simulink model "simulink_ros"  (R2022b)
settings: Solver=FixedStepAuto  StartTime=0.0  StopTime=setup.stop_time  FixedStep=setup.sim_ts  RelTol=1e-3
InitFcn:
  | %INIT_COSIM
StartFcn:
  | unix('source /home/pico/Documents/GitHub/bfmc/Simulator/devel/setup.bash; rosservice call /gazebo/reset_simulation');
undefined symbols (not defined in the file): nmpc_controller, setup
libraries: robotlib x5, simulink x2
settings Model: Creator=pico  LastModifiedBy=pico

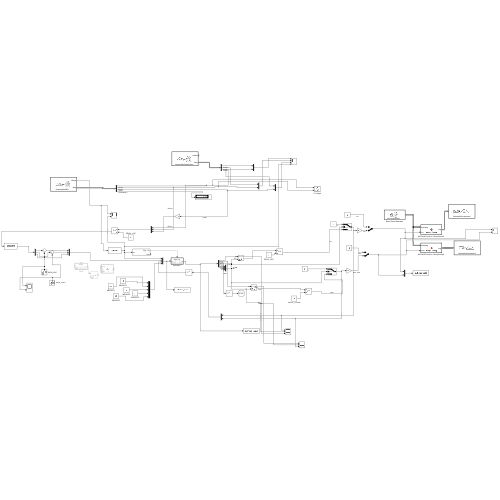
[thumbnail: Simulink's stored preview of the top-level diagram]
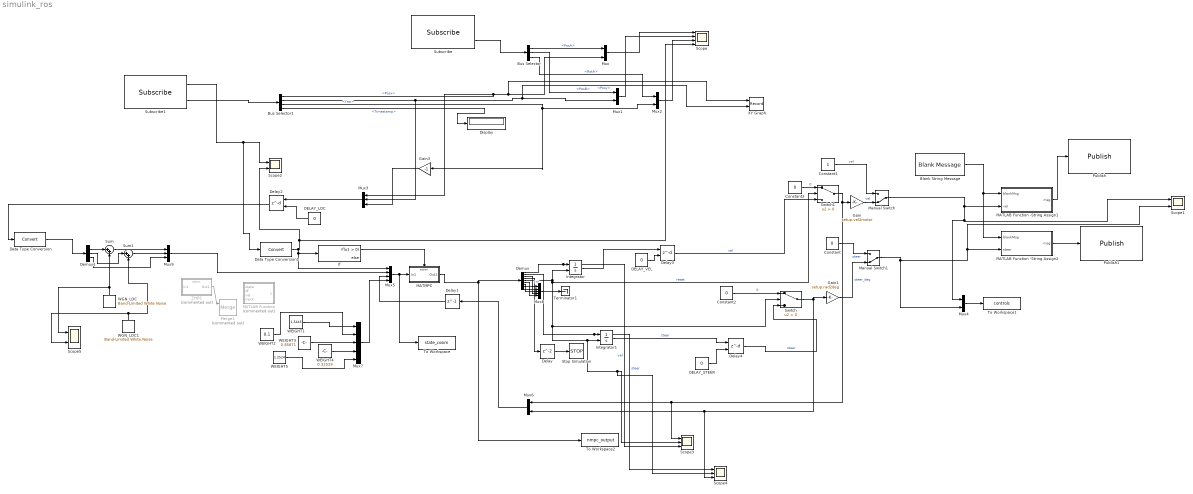
== system simulink_ros ==
  Blank String Message : robotlib/Blank Message  messageClass=Message  entityType=std_msgs/String  messageType=std_msgs/String  SampleTime=inf  legacyBusStruct=off
  Bus Selector : BusSelector  OutputSignals=PosA,PosB,RotA
  Bus Selector1 : BusSelector  OutputSignals=Posx,Posy,Yaw,Timestamp
  Constant : Constant  Value=0
  Constant1 : Constant
  Constant2 : Constant  Value=0
  Constant3 : Constant  Value=0
  DELAY_LOC : Constant  Value=0
  DELAY_STEER : Constant  Value=0
  DELAY_VEL : Constant  Value=0
  Data Type Conversion : DataTypeConversion  SaturateOnIntegerOverflow=off  RndMeth=Floor
  Data Type Conversion1 : DataTypeConversion  SaturateOnIntegerOverflow=off  RndMeth=Floor
  Delay : Delay
  Delay1 : Delay  DelayLength=1
  Delay2 : Delay  DelayLengthSource=Input port  DelayLength=0
      settings: InputPortMap=u0,p1
  Delay3 : Delay  DelayLengthSource=Input port  DelayLength=0
      settings: InputPortMap=u0,p1
  Delay4 : Delay  DelayLengthSource=Input port  DelayLength=0
      settings: InputPortMap=u0,p1
  Demux : Demux  Outputs=9
  Demux1 : Demux  Outputs=3
  Display : Display
  Gain : Gain  Gain=setup.vel2motor
  Gain1 : Gain  Gain=setup.rad2deg
  Gain3 : Gain  Gain=-1
  If : If
  Integrator : Integrator  ExternalReset=level  LimitOutput=on  UpperSaturationLimit=2  LowerSaturationLimit=0
  Integrator1 : Integrator  ExternalReset=level  LimitOutput=on  UpperSaturationLimit=pi/3  LowerSaturationLimit=-pi/3
  MATLAB Function : MATLAB Function  Commented=on  TreatAsAtomicUnit=on
  MATLAB Function -String Assign1 : MATLAB Function  TreatAsAtomicUnit=on
  MATLAB Function -String Assign2 : MATLAB Function  TreatAsAtomicUnit=on
  MATMPC : Subsystem  TreatAsAtomicUnit=on
  Manual Switch : ManualSwitch  CurrentSetting=0
  Manual Switch1 : ManualSwitch  CurrentSetting=0
  Merge1 : Merge  Commented=on
  Mux{,1..2,4,6} (5 alike) : Mux  Inputs=2
  Mux3 : Mux  Inputs=3
  Mux5 : Mux
  Mux7 : Mux  Inputs=5
  Mux8 : Mux  Inputs=5
  Mux9 : Mux  Inputs=3
  Publish : robotlib/Publish  topicSource=Select from ROS network  topic=/automobile/command  messageType=std_msgs/String  legacyBusStruct=off  messageQueueLength=1
      settings: LibrarySourceBlock=roslib/ROS/Publish
  Publish1 : robotlib/Publish  topicSource=Select from ROS network  topic=/automobile/command  messageType=std_msgs/String  legacyBusStruct=off  messageQueueLength=1
      settings: LibrarySourceBlock=roslib/ROS/Publish
  Scope : Scope  NumInputPorts=4
  Scope1 : Scope  NumInputPorts=2
  Scope2 : Scope  NumInputPorts=2
  Scope3 : Scope  NumInputPorts=3
  Scope4 : Scope  NumInputPorts=3
  Scope5 : Scope  NumInputPorts=2
  Stop Simulation : Stop
  Subscribe : robotlib/Subscribe  topicSource=Select from ROS network  topic=/automobile/localisation  messageType=utils/localisation  SampleTime=-1  legacyBusStruct=off  messageQueueLength=1
      settings: LibrarySourceBlock=roslib/ROS/Subscribe
  Subscribe1 : robotlib/Subscribe  topicSource=Select from ROS network  topic=/automobile/IMU  messageType=utils/IMU  SampleTime=-1  legacyBusStruct=off  messageQueueLength=1
      settings: LibrarySourceBlock=roslib/ROS/Subscribe
  Sum : Sum  Inputs=|++
  Sum1 : Sum  Inputs=|++
  Switch : Switch  Criteria=u2 > Threshold  SaturateOnIntegerOverflow=off  InputSameDT=off
  Switch1 : Switch  Criteria=u2 > Threshold  SaturateOnIntegerOverflow=off  InputSameDT=off
  Terminator1 : Terminator
  To Workspace : ToWorkspace  VariableName=state_cosim  SaveFormat=Structure With Time  SampleTime=-1
  To Workspace1 : ToWorkspace  VariableName=controls  SaveFormat=Structure With Time  SampleTime=-1
  To Workspace2 : ToWorkspace  VariableName=nmpc_output  SaveFormat=Structure With Time  SampleTime=-1
  WEIGHT1 : Constant  Value=1.5445
  WEIGHT2 : Constant  Value=0.1
  WEIGHT3 : Constant  Value=0.85671
  WEIGHT4 : Constant  Value=0.32529
  WEIGHT5 : Constant  Value=1.2524
  WGN_LOC : simulink/Sources/Band-Limited White Noise  Cov=WGN_LOC_PWR  Ts=setup.sim_ts  seed=[23341]
  WGN_LOC1 : simulink/Sources/Band-Limited White Noise  Cov=WGN_LOC_PWR  Ts=setup.sim_ts  seed=[23345]
  XY Graph : Record  FileSettingsInternal="{\"entries\":[{\"content\":{\"excelSettings\":{\"content\":{},\"type\":\"Streamout.ExcelSettings\"}},\"type\":\"Streamout.FileSettingStorage\",\"uuid\":\"7e36053c-6d87-4ba8-b961-ab87f153ee78\"}],\"packageUris\":[\"http://schema.mathworks.com/mf0/streamout_blocks/R2020a\"],\"version\":\"1.0\"}"  Layout=[1 1]  SignalsInternal="{\"entries\":[{\"content\":{\"signals\":[{\"content\":{\"blockPath\":[\"simulink_ros/XY Graph\"],\"channel\":[],\"dimensions\":[1],\"domain\":\"simulink_ros/XY Graph\",\"lineColor\":\"#a2142f\",\"plots\":[1],\"port\":1,\"sid\":[\"\"],\"signalID\":1424408,\"signalName\":\"<Posx>\"},\"type\":\"RecordBlkView.Signal\",\"uuid\":\"8700aef8-5ad9-478a-92a4-92141e58aa95\"},{\"content\":{\"blockPath\":[\"simulink_ros/XY Graph\"],\"channel\":[],\"dimensions\":[1],\"domain\":\"simulink_ros/XY Graph\",\"lineColor\":\"#139fff\",\"plots\":[1],\"port\":2,\"sid\":[\"\"],\"signalID\":1424412,\"signalName\":\"<Posy>\"},\"type\":\"RecordBlkView.Signal\",\"uuid\":\"c04be6e4-d870-4e8a-b9da-b27d68976f23\"}]},\"type\":\"RecordBlkView.InputSignals\",\"uuid\":\"eb864215-60c0-44ea-aa5a-99772fb5c421\"}],\"packageUris\":[\"http://schema.mathworks.com/mf0/streamout_blocks/R2020a\"],\"version\":\"1.0\"}"  VisualizationBindings="{\"xyplotplugin\":{\"info\":[{\"series\":[{\"bindingParametersList\":[{\"parameter\":\"X-Axis\",\"signalID\":1424408,\"signalName\":\"<Posx>\"},{\"parameter\":\"Y-Axis\",\"signalID\":1424412,\"signalName\":\"<Posy>\"}],\"seriesID\":29927}],\"subplotID\":1}]}}"  CompatibilityTag=XY
  ZHO1 : Subsystem  Commented=on  TreatAsAtomicUnit=on
  wires:
  Subscribe/2 -> Bus Selector/1
  Bus Selector/1 -> Mux/1  "<PosA>"
  Blank String Message/1 -> MATLAB Function -String Assign2/1(blankMsg), MATLAB Function -String Assign1/1(blankMsg)
  MATLAB Function -String Assign1/1(msg) -> Publish/1
  MATLAB Function -String Assign2/1(msg) -> Publish1/1
  Mux/1 -> Scope/1
  Bus Selector/2 -> Mux1/1  "<PosB>"
  Mux1/1 -> Scope/2
  Bus Selector/3 -> Mux2/1  "<RotA>"
  Mux2/1 -> Scope/3
  Bus Selector1/4 -> Display/1  "<Timestamp>"
  Bus Selector1/2 -> XY Graph/2, Mux1/2, Mux3/2  "<Posy>"
  Bus Selector1/3 -> Gain3/1, Mux2/2  "<Yaw>"
  Bus Selector1/1 -> Mux3/1, XY Graph/1, Mux/2  "<Posx>"
  Demux/2 -> Scope4/1, Integrator1/1  "steer"
  Demux/1 -> Scope3/3, Integrator/1  "vel"
  Manual Switch/1 -> Mux4/1, Scope1/1, MATLAB Function -String Assign1/2(vel)
  Constant1/1 -> Manual Switch/1  "vel"
  Constant/1 -> Manual Switch1/1  "steer"
  Manual Switch1/1 -> Mux4/2, Scope1/2, MATLAB Function -String Assign2/2(steer)
  Mux3/1 -> Delay2/1
  Demux/4 -> Delay/1
  Delay4/1 -> Switch/3  "steer"
  Mux4/1 -> To Workspace1/1
  Gain3/1 -> Mux3/3
  Data Type Conversion/1 -> Demux1/1
  Mux5/1 -> MATMPC/1(In1), To Workspace/1
  Integrator/1 -> Delay3/1
  Mux6/1 -> Delay1/1
  Switch/1 -> Scope4/3, Mux6/2, Gain1/1
  Switch1/1 -> Scope3/1, Mux6/1, Gain/1
  Delay3/1 -> Switch1/3  "vel"
  Constant2/1 -> Switch/1  "0"
  Constant3/1 -> Switch1/1  "0"
  Delay/1 -> Stop Simulation/1
  Subscribe1/1 -> Scope2/1, Data Type Conversion1/1
  Data Type Conversion1/1 -> If/1, Mux5/1, Scope/4, Scope2/2
  If/1 -> MATMPC/Action
  Delay1/1 -> Mux5/3
  MATMPC/1(Out1) -> To Workspace2/1, Demux/1
  ZHO1/1(Out1) -> Merge1/1
  Mux7/1 -> Mux5/4
  WEIGHT1/1 -> Mux7/1
  WEIGHT2/1 -> Mux7/2
  WEIGHT3/1 -> Mux7/3
  WEIGHT4/1 -> Mux7/4
  WEIGHT5/1 -> Mux7/5
  Demux/6 -> Mux8/2
  Demux/7 -> Mux8/3
  Demux/8 -> Mux8/4
  Demux/9 -> Mux8/5
  Demux/3 -> Mux8/1  "crv"
  Mux8/1 -> Terminator1/1
  Demux/5 -> Switch1/2, Switch/2, Scope4/2, Scope3/2, Integrator1/2, Integrator/2  "reset"
  Subscribe1/2 -> Bus Selector1/1
  DELAY_VEL/1 -> Delay3/2
  DELAY_STEER/1 -> Delay4/2
  DELAY_LOC/1 -> Delay2/2
  Delay2/1 -> Data Type Conversion/1
  Mux9/1 -> Mux5/2
  WGN_LOC/1 -> Sum/2, Scope5/1
  Demux1/1 -> Sum/1
  Sum/1 -> Mux9/1
  Sum1/1 -> Mux9/2
  Demux1/2 -> Sum1/1
  Demux1/3 -> Mux9/3
  WGN_LOC1/1 -> Sum1/2, Scope5/2
  Integrator1/1 -> Delay4/1  "steer"
  Gain1/1 -> Manual Switch1/2  "steer_deg"
  Gain/1 -> Manual Switch/2  "vel"

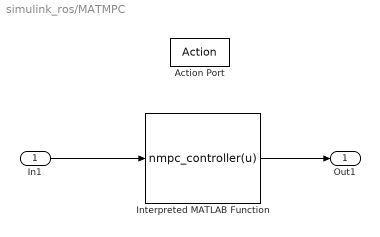
== system simulink_ros/MATMPC ==
  In1 : Inport
  Action Port : ActionPort  ActionPortLabel=if(u1 > 0)
  Interpreted MATLAB Function : MATLABFcn  MATLABFcn=nmpc_controller(u)  OutputDimensions=9
  Out1 : Outport
  wires:
  In1/1 -> Interpreted MATLAB Function/1
  Interpreted MATLAB Function/1 -> Out1/1

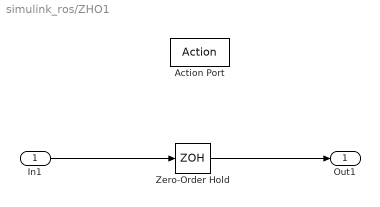
== system simulink_ros/ZHO1 ==
  In1 : Inport
  Action Port : ActionPort
  Zero-Order Hold : ZeroOrderHold  SampleTime=-1
  Out1 : Outport
  wires:
  In1/1 -> Zero-Order Hold/1
  Zero-Order Hold/1 -> Out1/1

== matlab function simulink_ros/MATLAB Function -String Assign2 ==
  data: blankMsg input; msg output Bus: SL_Bus_simulink_ros_std_msgs_String; steer input
function msg = assignString(blankMsg,steer)
% assignString - Assign a string in a ROS message
%
% MSG = assignString(blankMsg) assigns a known string value to a 
%  string field in a ROS message, and outputs the updated ROS message.
%
%  blankMsg (input): A bus for a 'std_msgs/String' message. This is 
%      used to initialize the output. 
%  msg (output): A bus for a 'std_msgs/String' message, with the Data 
%      field set to a string.

%   Copyright 2015 The MathWorks, Inc.
%#codegen

% Note: The datatype of 'msg' has been explicitly set to the appropriate 
% Simulink bus type ("Bus: SL_Bus_robotROSMessageUsageExample_std_msgs_String"). 
%
% If the model name is changed, the datatype needs to be changed as well:
%   1) Click "Edit Data" in the Editor toolstrip to open "Ports and Data Manager"
%   2) Select "msg". From the "Type" dropdown, select "--- Refresh data types ---"
%   3) Set datatype to "Bus: SL_Bus_<modelname>_std_msgs_String"
    
% stringToAssign = 'information';
steer_string = sprintf('%.1f',steer);
% "{\"action\": \"1\", \"speed\": -0.1}"
stringToAssign = ['{"action": "2", "steerAngle": ',steer_string,'}'];%['action\', '1', 'speed',u];

msg = blankMsg;

% msg (std_msgs/String) consists of
%           Data : array of type uint8
%   Data_SL_Info : struct with fields CurrentLength, ReceivedLength
strLength = length(stringToAssign);
msg.Data(1:strLength) = uint8(stringToAssign);
msg.Data_SL_Info.CurrentLength = uint32(strLength);

== matlab function simulink_ros/MATLAB Function ==
  data: state input; y output; df input; vel input; input input
function y = fcn(state,df,vel,input)

X = state(1);
Y = state(2);
PSI = state(3);

% l_r = input.od(2,1);
% l_f = input.od(3,1);
% 
% beta = atan(l_r/(l_f+l_r)*tan(d));

% velocities
% vx = v*cos(beta+PSI); % local
vx = v*cos(PSI); % local

y = [X;Y;PSI;vx;df];

== matlab function simulink_ros/MATLAB Function -String Assign1 ==
  data: blankMsg input; msg output Bus: SL_Bus_simulink_ros_std_msgs_String; vel input
function msg = assignString(blankMsg,vel)
% assignString - Assign a string in a ROS message
%
% MSG = assignString(blankMsg) assigns a known string value to a 
%  string field in a ROS message, and outputs the updated ROS message.
%
%  blankMsg (input): A bus for a 'std_msgs/String' message. This is 
%      used to initialize the output. 
%  msg (output): A bus for a 'std_msgs/String' message, with the Data 
%      field set to a string.

%   Copyright 2015 The MathWorks, Inc.
%#codegen

% Note: The datatype of 'msg' has been explicitly set to the appropriate 
% Simulink bus type ("Bus: SL_Bus_robotROSMessageUsageExample_std_msgs_String"). 
%
% If the model name is changed, the datatype needs to be changed as well:
%   1) Click "Edit Data" in the Editor toolstrip to open "Ports and Data Manager"
%   2) Select "msg". From the "Type" dropdown, select "--- Refresh data types ---"
%   3) Set datatype to "Bus: SL_Bus_<modelname>_std_msgs_String"
    
thr_string = sprintf('%.1f',vel);
% "{\"action\": \"1\", \"speed\": -0.1}"
stringToAssign = ['{"action": "1", "speed": ',thr_string,'}'];%['action\', '1', 'speed',u];

msg = blankMsg;

% msg (std_msgs/String) consists of
%           Data : array of type uint8
%   Data_SL_Info : struct with fields CurrentLength, ReceivedLength
strLength = length(stringToAssign);
msg.Data(1:strLength) = uint8(stringToAssign);
msg.Data_SL_Info.CurrentLength = uint32(strLength);
